simulink model "day10p1"  (R2026a)
settings: Solver=FixedStepDiscrete  StopTime=inf
InitFcn:
  | % lmpCntMax = 6;
  | lmpCntMax = 10;
  | % btnCntMax = 10;
  | btnCntMax = 16;
  | % btnStrMax = 39;
  | btnStrMax = 181;
  | lmpStrMax = lmpCntMax + 2;
  | possibilities = dec2bin([0:((2^btnCntMax) - 1)]) - '0';
  | [~, ixs] = sort(sum(possibilities, 2));
  | possibilities = possibilities(ixs, :);
undefined symbols (not defined in the file): DiscIntNeverNeededParam
libraries: simulink x5
(part 2 of 2)

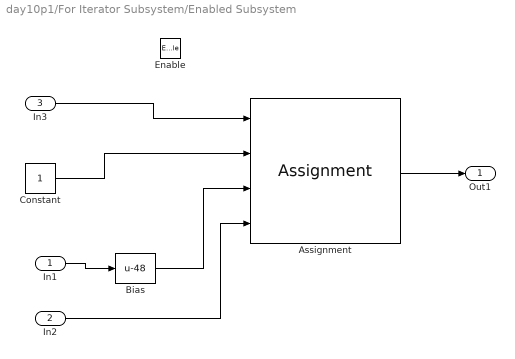
== system day10p1/For Iterator Subsystem/Enabled Subsystem ==
  In1 : Inport
  In2 : Inport  Port=2
  In3 : Inport  Port=3
  Enable : EnablePort  StatesWhenEnabling=reset
  Assignment : Assignment  NumberOfDimensions=2  IndexMode=Zero-based  DiagnosticForDimensions=Warning  IndexOptions=Index vector (port),Index vector (port)  Indices=1,1  OutputSizes=1,1  RuntimeRangeChecks=on
  Bias : Bias  Bias=-48  SaturateOnIntegerOverflow=off
  Constant : Constant
  Out1 : Outport
  wires:
  In1/1 -> Bias/1
  In3/1 -> Assignment/1
  Constant/1 -> Assignment/2
  Bias/1 -> Assignment/3
  In2/1 -> Assignment/4
  Assignment/1 -> Out1/1
